simulink model "matchedfilter"  (Simulink 10.3)
settings: Solver=VariableStepAuto  StartTime=0.0  StopTime=1000.0  RelTol=1e-3
libraries: dsp_blocks x7
settings Model: Creator=nathanalemayehu  LastModifiedBy=nathanalemayehu
settings SolverCC: AlgebraicLoopSolver=Auto
settings DataIOCC: SaveFormat=Dataset  SignalLoggingSaveFormat=Dataset  ReturnWorkspaceOutputs=on
settings OptimizationCC: ExpressionDepthLimit=128  LifeSpan=auto
settings DebuggingCC: UnderspecifiedInitializationDetection=Simplified  MergeDetectMultiDrivingBlocksExec=error  FcnCallInpInsideContextMsg=error  StateNameClashWarn=none  SFUnexpectedBacktrackingDiag=error  SFNoUnconditionalDefaultTransitionDiag=error  SFExecutionAtInitializationDiag=warning  SFMachineParentedDataDiag=error  ArithmeticOperatorsInVariantConditions=error
settings HardwareCC: ProdBitPerPointer=64  ProdBitPerSizeT=64  ProdBitPerPtrDiffT=64  ProdLargestAtomicFloat=Float  ProdIntDivRoundTo=Zero  ProdEndianess=LittleEndian  ProdWordSize=64  ProdHWDeviceType=Intel->x86-64 (Windows64)
settings ModelReferenceCC: PropagateSignalLabelsOutOfModel=on
settings SFSimCC: SimUseLocalCustomCode=on  CustomCodeUndefinedFunction=FilterOut
settings RTWCC: RTWUseLocalCustomCode=on
settings CodeAppCC: StateflowObjectComments=off
settings GRTTargetCC: TargetLangStandard=C99 (ISO)  CombineOutputUpdateFcns=on  GRTInterface=off
settings ConfigComp: CovMetricSettings=dwe  CovSaveCumulativeToWorkspaceVar=off  CovSaveSingleToWorkspaceVar=off  CovExternalEMLEnable=on

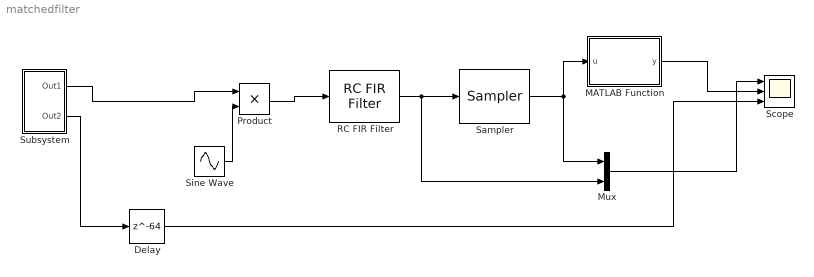
== system matchedfilter ==
  Delay : Delay  DelayLength=64
  MATLAB Function : MATLAB Function  TreatAsAtomicUnit=on
  Mux : Mux  Inputs=2
  Product : Product
  RC FIR Filter : dsp_blocks/Filters/RC FIR Filter  period=50  beta=0.5  root=off  filt_len=128  win_type=on
  Sampler : dsp_blocks/Conversions/Sampler  offset=80  samp_period=50
  Scope : Scope  NumInputPorts=3
  Sine Wave : Sin  Amplitude=2  Frequency=2*pi*0.1  SampleTime=0
  Subsystem : Subsystem
  wires:
  Subsystem/2(Out2) -> Delay/1
  Sine Wave/1 -> Product/2
  Subsystem/1(Out1) -> Product/1
  Mux/1 -> Scope/1
  MATLAB Function/1(y) -> Scope/2
  Delay/1 -> Scope/3
  RC FIR Filter/1 -> Mux/2, Sampler/1
  Sampler/1 -> MATLAB Function/1(u), Mux/1
  Product/1 -> RC FIR Filter/1

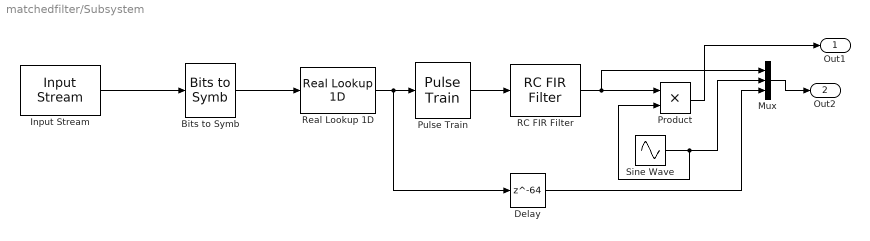
== system matchedfilter/Subsystem ==
  Bits to Symb : dsp_blocks/Conversions/Bits to Symb
  Delay : Delay  DelayLength=64
  Input Stream : dsp_blocks/Sources//Sinks/Input Stream  period=50  width=1  fname=rand.mat
  Mux : Mux  Inputs=3
  Product : Product
  Pulse Train : dsp_blocks/Conversions/Pulse Train  period=50
  RC FIR Filter : dsp_blocks/Filters/RC FIR Filter  period=50  beta=0.5  root=off  filt_len=128  win_type=on
  Real Lookup 1D : dsp_blocks/Conversions/Real Lookup 1D  table=[-1 1]
  Sine Wave : Sin  Frequency=2*pi*0.1  SampleTime=0
  Out1 : Outport
  Out2 : Outport  Port=2
  wires:
  Input Stream/1 -> Bits to Symb/1
  Bits to Symb/1 -> Real Lookup 1D/1
  Product/1 -> Out1/1
  Sine Wave/1 -> Mux/2, Product/2
  Pulse Train/1 -> RC FIR Filter/1
  Mux/1 -> Out2/1
  Real Lookup 1D/1 -> Delay/1, Pulse Train/1
  Delay/1 -> Mux/3
  RC FIR Filter/1 -> Mux/1, Product/1

== matlab function MATLAB Function ==
  data: u input double; y output double
function y = fcn(u)
if(u > 0),
    y = 1;
else 
    y = 0;
end
